simulink model "trab2_model4"  (Simulink 7.6)
settings: Solver=VariableStepDiscrete  SolverMode=SingleTasking  StartTime=0.0  StopTime=10  FixedStep=1/100000  RelTol=1e-3  AbsTol=1e-6
PreLoadFcn:
  | M=16;
libraries: commutil2 x2, commsink2 x2, commdigbbndam3 x2, commchan3 x1, commrandsrc2 x1
settings Model: Creator=amoura  LastModifiedBy=Sílvio
settings DataIOCC: LimitDataPoints=off
settings OptimizationCC: BlockReduction=off  BooleanDataType=off  InitFltsAndDblsToZero=on
settings DebuggingCC: SaveWithParameterizedLinksMsg=none  SignalResolutionControl=TryResolveAllWithWarning  SolverPrmCheckMsg=none  MultiTaskDSMMsg=warning  MultiTaskCondExecSysMsg=none  StrictBusMsg=None
settings HardwareCC: TargetUnknown=on
settings RTWCC: TemplateMakefile=grt_unix.tmf  IncludeERTFirstTime=on
settings GRTTargetCC: TargetFcnLib=ansi_tfl_tmw.mat  ModelReferenceCompliant=off  MatFileLogging=off

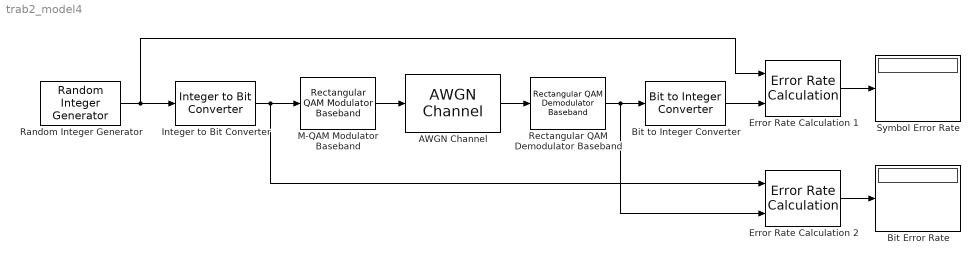
== system trab2_model4 ==
  AWGN Channel : commchan3/AWGN Channel  SystemSampleTime=-1  InputProcessing=Columns as channels (frame based)  seed=67  noiseMode="Signal to noise ratio  (Es/No)"  EbNodB=9.21  EsNodB=8  SNRdB=10  bitsPerSym=3  Ps=1  Tsym=1/1000  variance=1
  Bit Error Rate : Display
  Bit to Integer Converter : commutil2/Bit to Integer Converter  nbits=log2(M)  bitOrder=MSB first  signedOutputValues=Unsigned  outDtype=Inherit via internal rule  outDtypeSigned=Inherit via internal rule
  Error Rate Calculation 1 : commsink2/Error Rate Calculation  N=0  st_delay=0  cp_mode=Entire frame  subframe=[]  PMode=Port  WsName=ErrorVec  RsMode2=off  stop=off  numErr=100  maxBits=1e6
  Error Rate Calculation 2 : commsink2/Error Rate Calculation  N=0  st_delay=0  cp_mode=Entire frame  subframe=[]  PMode=Port  WsName=ErrorVec  RsMode2=off  stop=off  numErr=100  maxBits=1e6
  Integer to Bit Converter : commutil2/Integer to Bit Converter  nbits=log2(M)  signedInputValues=Unsigned  bitOrder=MSB first  outDtype=Inherit via internal rule
  M-QAM Modulator Baseband : commdigbbndam3/Rectangular QAM Modulator Baseband  DialogController=commDDGCreate  DialogControllerArgs=DataTag1  M=M  InType=Bit  Enc=Gray  Mapping=[0:15]  PowType=Min. distance between symbols  MinDist=0.7  AvgPow=1  PeakPow=1  Ph=0  outDtype=double  outWordLen=16  outUDDataType=sfix(16)  outFracLenMode=Best precision  outFracLen=15
  Random Integer Generator : commrandsrc2/Random Integer Generator  SystemSampleTime=-1  mul=M  seed=529510  Ts=1/1000  frameBased=on  sampPerFrame=100  orient=off  outDataType=double
  Rectangular QAM Demodulator Baseband : commdigbbndam3/Rectangular QAM Demodulator Baseband  DialogController=commDDGCreate  DialogControllerArgs=DataTag2  M=M  PowType=Min. distance between symbols  MinDist=0.7  AvgPow=1  PeakPow=1  Ph=0  Dec=Gray  Mapping=[0:15]  OutType=Bit  DecType=Hard decision  VarSource=Dialog  Variance=1  outDtype1=Inherit via internal rule  outDtype2=Inherit via internal rule  derotateFactorWordLen=16  denormFactorWordLen=16  prodOutWordLen=32  prodOutRoundingMode=Floor  prodOutOverflowMode=Wrap  sumWordLen=32
  "Symbol Error Rate " : Display
  wires:
  Error Rate Calculation 1/1 -> "Symbol Error Rate "/1
  Random Integer Generator/1 -> Error Rate Calculation 1/1, Integer to Bit Converter/1
  AWGN Channel/1 -> Rectangular QAM Demodulator Baseband/1
  M-QAM Modulator Baseband/1 -> AWGN Channel/1
  Integer to Bit Converter/1 -> Error Rate Calculation 2/1, M-QAM Modulator Baseband/1
  Rectangular QAM Demodulator Baseband/1 -> Bit to Integer Converter/1, Error Rate Calculation 2/2
  Bit to Integer Converter/1 -> Error Rate Calculation 1/2
  Error Rate Calculation 2/1 -> Bit Error Rate/1
